simulink subsystem "DC_Gearbox_Motor"  (R2024b)
settings: Solver=VariableStepAuto  StartTime=0.0  StopTime=10.0  RelTol=1e-3
undefined symbols (not defined in the file or in its folder): Beq, Jeq, Ke, Kt, La, n, Ra
settings Model: Creator=rodrigoscott  LastModifiedBy=rodrigoscott

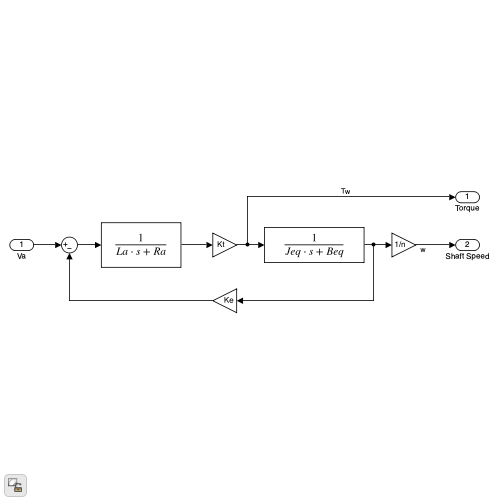
[thumbnail: Simulink's stored preview of the top-level diagram]
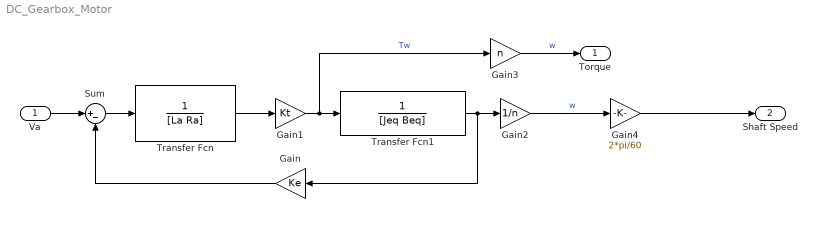
== system DC_Gearbox_Motor ==
  Va : Inport
  Gain : Gain  Gain=Ke
  Gain1 : Gain  Gain=Kt
  Gain2 : Gain  Gain=1/n
  Gain3 : Gain  Gain=n
  Gain4 : Gain  Gain=2*pi/60
  Sum : Sum  Inputs=|+-
  Transfer Fcn : TransferFcn  Denominator=[La Ra]
  Transfer Fcn1 : TransferFcn  Denominator=[Jeq Beq]
  Torque : Outport
  Shaft Speed : Outport  Port=2
  wires:
  Transfer Fcn/1 -> Gain1/1
  Gain/1 -> Sum/2
  Gain2/1 -> Gain4/1  "w"
  Sum/1 -> Transfer Fcn/1
  Gain1/1 -> Transfer Fcn1/1, Gain3/1  "Tw"
  Va/1 -> Sum/1
  Transfer Fcn1/1 -> Gain2/1, Gain/1
  Gain3/1 -> Torque/1  "w"
  Gain4/1 -> Shaft Speed/1
